simulink model "sigma_delta"  (R2014a)
settings: Solver=ode45  StartTime=0.0  StopTime=inf  RelTol=1e-3
values from neighbouring files (symbols this model uses):
  SampleTime = 3.25520833333e-06    [sigma-delta.mat]
undefined symbols (not defined in the file or in its folder): C, R
libraries: simulink_extras x2, dspsigops x2, simulink x1
settings Model: Creator=root  LastModifiedBy=root

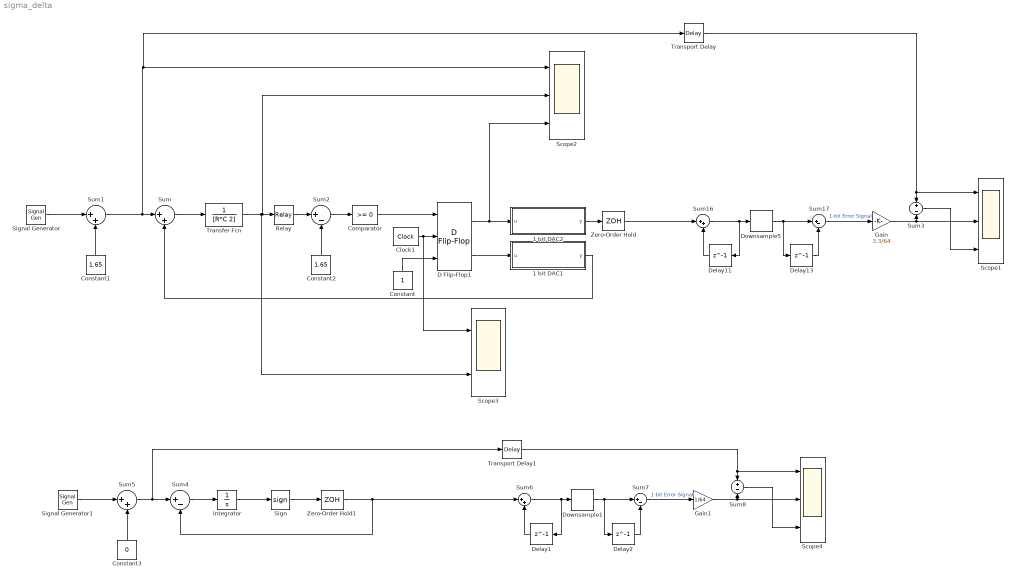
== system sigma_delta ==
  1 bit DAC1 : MATLAB Function  TreatAsAtomicUnit=on
  1 bit DAC2 : MATLAB Function  TreatAsAtomicUnit=on
  Clock1 : simulink_extras/Flip Flops/Clock  period=SampleTime
  Comparator : simulink/Logic and Bit Operations/Compare To Zero  relop=>=  OutDataTypeStr=boolean  ZeroCross=off
  Constant : Constant  SampleTime=0
  Constant1 : Constant  Value=1.65  SampleTime=0
  Constant2 : Constant  Value=1.65  SampleTime=0
  Constant3 : Constant  Value=0  SampleTime=0
  D Flip-Flop1 : simulink_extras/Flip Flops/D Flip-Flop
  Delay1 : Delay  DelayLength=1  SampleTime=SampleTime
  Delay11 : Delay  DelayLength=1  SampleTime=SampleTime
  Delay13 : Delay  DelayLength=1  SampleTime=64*SampleTime
  Delay2 : Delay  DelayLength=1  SampleTime=64*SampleTime
  Downsample1 : dspsigops/Downsample  N=64  phase=0  RateOptions=Allow multirate processing  smode=Allow multirate  fmode=Maintain input frame size  ic=0
  Downsample5 : dspsigops/Downsample  N=64  phase=0  RateOptions=Allow multirate processing  smode=Allow multirate  fmode=Maintain input frame size  ic=0
  Gain : Gain  Gain=3.3/64
  Gain1 : Gain  Gain=1/64
  Integrator : Integrator
  Relay : Relay  OnSwitchValue=1.65  OffSwitchValue=1.65  OnOutputValue=3.3
  Scope1 : Scope  NumInputPorts=3
      settings: TimeRange=0.125  YMin=0.6~0.6~-0.2  YMax=2.7~2.7~0.2
  Scope2 : Scope  NumInputPorts=3
      settings: TimeRange=0.125  YMin=0.6~1.595~0  YMax=2.7~1.705~1
  Scope3 : Scope  NumInputPorts=2
      settings: TimeRange=0.0003  YMin=0.0027625~0.1855  YMax=0.00282~0.1874  SaveName=ScopeData2
  Scope4 : Scope  NumInputPorts=3
      settings: TimeRange=0.125  YMin=-1~-1~-0.175  YMax=1~1~0.175  SaveName=ScopeData3
  Sign : Signum
  Signal Generator : SignalGenerator  Frequency=20
  Signal Generator1 : SignalGenerator  Frequency=20
  Sum{,1,5..6,16} (5 alike) : Sum  Inputs=|++
  Sum{2,4,7,17} (4 alike) : Sum  Inputs=|+-
  Sum3 : Sum  Inputs=+|-
  Sum8 : Sum  Inputs=+|-
  Transfer Fcn : TransferFcn  Denominator=[R*C 2]
  Transport Delay : TransportDelay  DelayTime=64*3/512000
  Transport Delay1 : TransportDelay  DelayTime=64*3/512000
  Zero-Order Hold : ZeroOrderHold  SampleTime=SampleTime
  Zero-Order Hold1 : ZeroOrderHold  SampleTime=SampleTime
  wires:
  Delay11/1 -> Sum16/2
  Sum16/1 -> Delay11/1, Downsample5/1
  Delay13/1 -> Sum17/2
  Downsample5/1 -> Sum17/1, Delay13/1
  Sum/1 -> Transfer Fcn/1
  Constant/1 -> D Flip-Flop1/3
  Clock1/1 -> Scope3/1, D Flip-Flop1/2
  D Flip-Flop1/2 -> 1 bit DAC1/1(u)
  1 bit DAC1/1(y) -> Sum/2
  Transfer Fcn/1 -> Scope2/2, Relay/1, Scope3/2
  D Flip-Flop1/1 -> Scope2/3, 1 bit DAC2/1(u)
  Zero-Order Hold/1 -> Sum16/1
  1 bit DAC2/1(y) -> Zero-Order Hold/1
  Comparator/1 -> D Flip-Flop1/1
  Signal Generator/1 -> Sum1/1
  Constant1/1 -> Sum1/2
  Sum17/1 -> Gain/1  "1-bit Error Signal"
  Constant2/1 -> Sum2/2
  Relay/1 -> Sum2/1
  Sum2/1 -> Comparator/1
  Gain/1 -> Sum3/2, Scope1/2
  Sum3/1 -> Scope1/3
  Sum1/1 -> Sum/1, Transport Delay/1, Scope2/1
  Transport Delay/1 -> Scope1/1, Sum3/1
  Integrator/1 -> Sign/1
  Sign/1 -> Zero-Order Hold1/1
  Sum4/1 -> Integrator/1
  Signal Generator1/1 -> Sum5/1
  Constant3/1 -> Sum5/2
  Sum5/1 -> Transport Delay1/1, Sum4/1
  Delay1/1 -> Sum6/2
  Sum6/1 -> Delay1/1, Downsample1/1
  Delay2/1 -> Sum7/2
  Downsample1/1 -> Sum7/1, Delay2/1
  Zero-Order Hold1/1 -> Sum4/2, Sum6/1
  Sum7/1 -> Gain1/1  "1-bit Error Signal"
  Gain1/1 -> Sum8/2, Scope4/2
  Sum8/1 -> Scope4/3
  Transport Delay1/1 -> Scope4/1, Sum8/1

== matlab function sigma_delta/1 bit DAC1 ==
  data: u input; y output
function y = DAC_1_bit(u)
% This block supports an embeddable subset of the MATLAB language.
% See the help menu for details.

% This code converts boolean input to a bipolar output (double precision).
% We chose to write this in EML function block but we could have also done 
% this with simulink blocks.

y=3.3*u;

== matlab function sigma_delta/1 bit DAC2 ==
  data: u input; y output
function y = DAC_1_bit(u)
% This block supports an embeddable subset of the MATLAB language.
% See the help menu for details.

% This code converts boolean input to a bipolar output (double precision).
% We chose to write this in EML function block but we could have also done 
% this with simulink blocks.

y=1*u;
